simulink model "lab1model"  (R2021a)
settings: Solver=VariableStepAuto  StartTime=0.0  StopTime=10.0  RelTol=1e-3
settings Model: Creator=ajendo  LastModifiedBy=ajendo

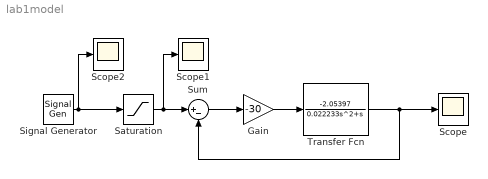
== system lab1model ==
  Gain : Gain  Gain=-30
  Saturation : Saturate  UpperLimit=0.7  LowerLimit=-0.7
  Scope : Scope
  Scope1 : Scope
  Scope2 : Scope
  Signal Generator : SignalGenerator  WaveForm=square  Amplitude=2  Units=rad/sec
  Sum : Sum  Inputs=|+-
  Transfer Fcn : TransferFcn  Numerator=[-2.05397]  Denominator=[0.022233 1 0]
  wires:
  Gain/1 -> Transfer Fcn/1
  Transfer Fcn/1 -> Sum/2, Scope/1
  Saturation/1 -> Scope1/1, Sum/1
  Sum/1 -> Gain/1
  Signal Generator/1 -> Scope2/1, Saturation/1
